simulink model "lab02_Digital_Inputs_and_Outputs"  (R2022b)
settings: Solver=FixedStepAuto  StartTime=0.0  StopTime=inf  RelTol=1e-3
libraries: arduinolib x10, simulink x6
settings Model: ExtModeTrigDuration=2  Creator=MAAM  LastModifiedBy=MAAM
settings OptimizationCC: EnhancedBackFolding=on  PassReuseOutputArgsAs=Individual arguments  ZeroExternalMemoryAtStartup=off  ZeroInternalMemoryAtStartup=off  MaxStackSize=64  OptimizeBlockOrder=speed  DifferentSizesBufferReuse=on  OptimizationCustomize=off  EfficientTunableParamExpr=on
settings DebuggingCC: ParameterTunabilityLossMsg=error
settings HardwareCC: ProdBitPerInt=16  ProdBitPerPointer=16  ProdBitPerSizeT=16  ProdBitPerPtrDiffT=16  ProdLargestAtomicFloat=None  ProdWordSize=8  ProdHWDeviceType=Atmel->AVR
settings SFSimCC: MATLABDynamicMemAlloc=off
settings RTWCC: Description=Embedded Coder  SystemTargetFile=ert.tlc  HardwareBoard=Arduino Mega 2560  TemplateMakefile=ert_default_tmf  Toolchain=Arduino AVR  BuildConfiguration=Faster Runs
settings CodeAppCC: ForceParamTrailComments=on  IgnoreCustomStorageClasses=off  OperatorAnnotations=on  SimulinkDataObjDesc=on  SFDataObjDesc=on  InsertBlockDesc=on
settings ERTTargetCC: SupportContinuousTime=on  SupportVariableSizeSignals=on  ExtMode=on  ExtModeTransport=3  ExtModeStaticAlloc=on  ExtModeAutomaticAllocSize=off  ExtModeStaticAllocSize=2048  ExtModeMexFile=ext_xcp  ExtModeMexArgs=0 5 921600  ExtModeIntrfLevel=Level2 - Open

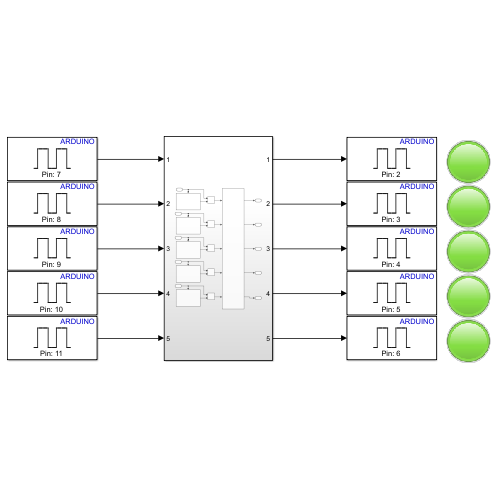
[thumbnail: Simulink's stored preview of the top-level diagram]
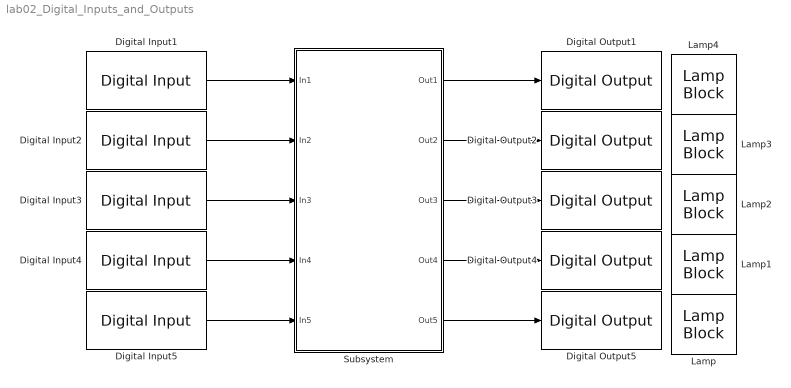
== system lab02_Digital_Inputs_and_Outputs ==
  Digital Input1 : arduinolib/Digital Input  pinNumber=7  mode=Default  Direction=input  SampleTime=-1  blockPlatform=arduino
  Digital Input2 : arduinolib/Digital Input  pinNumber=8  mode=Default  Direction=input  SampleTime=-1  blockPlatform=arduino
  Digital Input3 : arduinolib/Digital Input  pinNumber=9  mode=Default  Direction=input  SampleTime=-1  blockPlatform=arduino
  Digital Input4 : arduinolib/Digital Input  pinNumber=10  mode=Default  Direction=input  SampleTime=-1  blockPlatform=arduino
  Digital Input5 : arduinolib/Digital Input  pinNumber=11  mode=Default  Direction=input  SampleTime=-1  blockPlatform=arduino
  Digital Output1 : arduinolib/Digital Output  pinNumber=2  Direction=output  blockPlatform=arduino
  Digital Output2 : arduinolib/Digital Output  pinNumber=3  Direction=output  blockPlatform=arduino
  Digital Output3 : arduinolib/Digital Output  pinNumber=4  Direction=output  blockPlatform=arduino
  Digital Output4 : arduinolib/Digital Output  pinNumber=5  Direction=output  blockPlatform=arduino
  Digital Output5 : arduinolib/Digital Output  pinNumber=6  Direction=output  blockPlatform=arduino
  Lamp{,1..4} (5 alike) : LampBlock  LabelPosition=Hide
  Subsystem : Subsystem
  wires:
  Subsystem/4(Out4) -> Digital Output4/1
  Subsystem/3(Out3) -> Digital Output3/1
  Subsystem/2(Out2) -> Digital Output2/1
  Subsystem/1(Out1) -> Digital Output1/1
  Digital Input1/1 -> Subsystem/1(In1)
  Digital Input2/1 -> Subsystem/2(In2)
  Digital Input3/1 -> Subsystem/3(In3)
  Digital Input4/1 -> Subsystem/4(In4)
  Digital Input5/1 -> Subsystem/5(In5)
  Subsystem/5(Out5) -> Digital Output5/1

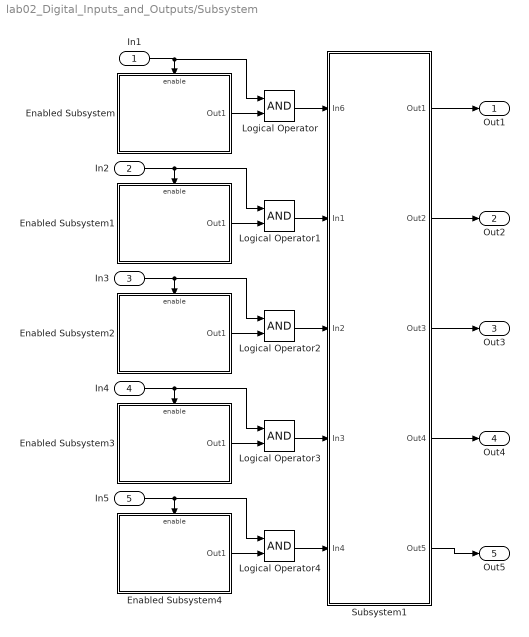
== system lab02_Digital_Inputs_and_Outputs/Subsystem ==
  In1 : Inport
  In2 : Inport  Port=2
  In3 : Inport  Port=3
  In4 : Inport  Port=4
  In5 : Inport  Port=5
  Enabled Subsystem : Subsystem  TreatAsAtomicUnit=on
  Enabled Subsystem1 : Subsystem  TreatAsAtomicUnit=on
  Enabled Subsystem2 : Subsystem  TreatAsAtomicUnit=on
  Enabled Subsystem3 : Subsystem  TreatAsAtomicUnit=on
  Enabled Subsystem4 : Subsystem  TreatAsAtomicUnit=on
  Logical Operator{,1..4} (5 alike) : Logic  AllPortsSameDT=off  OutDataTypeStr=boolean
  Subsystem1 : Subsystem
  Out1 : Outport
  Out2 : Outport  Port=2
  Out3 : Outport  Port=3
  Out4 : Outport  Port=4
  Out5 : Outport  Port=5
  wires:
  In1/1 -> Logical Operator/1, Enabled Subsystem/Enable
  In2/1 -> Logical Operator1/1, Enabled Subsystem1/Enable
  In3/1 -> Enabled Subsystem2/Enable, Logical Operator2/1
  In4/1 -> Logical Operator3/1, Enabled Subsystem3/Enable
  In5/1 -> Logical Operator4/1, Enabled Subsystem4/Enable
  Enabled Subsystem/1(Out1) -> Logical Operator/2
  Enabled Subsystem1/1(Out1) -> Logical Operator1/2
  Enabled Subsystem2/1(Out1) -> Logical Operator2/2
  Enabled Subsystem3/1(Out1) -> Logical Operator3/2
  Enabled Subsystem4/1(Out1) -> Logical Operator4/2
  Subsystem1/5(Out5) -> Out5/1
  Subsystem1/4(Out4) -> Out4/1
  Subsystem1/3(Out3) -> Out3/1
  Subsystem1/2(Out2) -> Out2/1
  Subsystem1/1(Out1) -> Out1/1
  Logical Operator4/1 -> Subsystem1/5(In4)
  Logical Operator3/1 -> Subsystem1/4(In3)
  Logical Operator2/1 -> Subsystem1/3(In2)
  Logical Operator1/1 -> Subsystem1/2(In1)
  Logical Operator/1 -> Subsystem1/1(In6)

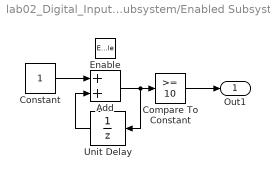
== system lab02_Digital_Inputs_and_Outputs/Subsystem/Enabled Subsystem ==
  Enable : EnablePort  StatesWhenEnabling=reset
  Add : Sum
  Compare To Constant : simulink/Logic and Bit Operations/Compare To Constant  relop=>=  const=10  OutDataTypeStr=boolean
  Constant : Constant
  Unit Delay : UnitDelay  SampleTime=0.1  HasFrameUpgradeWarning=on
  Out1 : Outport
  wires:
  Add/1 -> Compare To Constant/1, Unit Delay/1
  Unit Delay/1 -> Add/2
  Constant/1 -> Add/1
  Compare To Constant/1 -> Out1/1

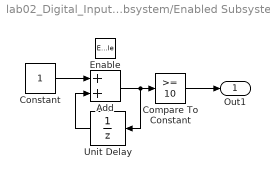
== system lab02_Digital_Inputs_and_Outputs/Subsystem/Enabled Subsystem1 ==
  Enable : EnablePort  StatesWhenEnabling=reset
  Add : Sum
  Compare To Constant : simulink/Logic and Bit Operations/Compare To Constant  relop=>=  const=10  OutDataTypeStr=boolean
  Constant : Constant
  Unit Delay : UnitDelay  SampleTime=0.1  HasFrameUpgradeWarning=on
  Out1 : Outport
  wires:
  Compare To Constant/1 -> Out1/1
  Constant/1 -> Add/1
  Unit Delay/1 -> Add/2
  Add/1 -> Unit Delay/1, Compare To Constant/1

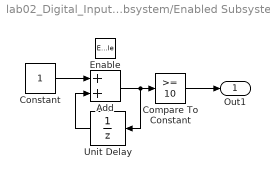
== system lab02_Digital_Inputs_and_Outputs/Subsystem/Enabled Subsystem2 ==
  Enable : EnablePort  StatesWhenEnabling=reset
  Add : Sum
  Compare To Constant : simulink/Logic and Bit Operations/Compare To Constant  relop=>=  const=10  OutDataTypeStr=boolean
  Constant : Constant
  Unit Delay : UnitDelay  SampleTime=0.1  HasFrameUpgradeWarning=on
  Out1 : Outport
  wires:
  Add/1 -> Compare To Constant/1, Unit Delay/1
  Unit Delay/1 -> Add/2
  Constant/1 -> Add/1
  Compare To Constant/1 -> Out1/1

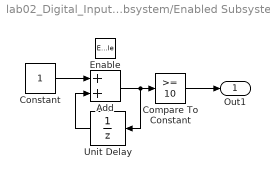
== system lab02_Digital_Inputs_and_Outputs/Subsystem/Enabled Subsystem3 ==
  Enable : EnablePort  StatesWhenEnabling=reset
  Add : Sum
  Compare To Constant : simulink/Logic and Bit Operations/Compare To Constant  relop=>=  const=10  OutDataTypeStr=boolean
  Constant : Constant
  Unit Delay : UnitDelay  SampleTime=0.1  HasFrameUpgradeWarning=on
  Out1 : Outport
  wires:
  Compare To Constant/1 -> Out1/1
  Constant/1 -> Add/1
  Unit Delay/1 -> Add/2
  Add/1 -> Unit Delay/1, Compare To Constant/1

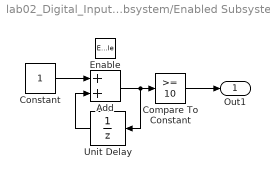
== system lab02_Digital_Inputs_and_Outputs/Subsystem/Enabled Subsystem4 ==
  Enable : EnablePort  StatesWhenEnabling=reset
  Add : Sum
  Compare To Constant : simulink/Logic and Bit Operations/Compare To Constant  relop=>=  const=10  OutDataTypeStr=boolean
  Constant : Constant
  Unit Delay : UnitDelay  SampleTime=0.1  HasFrameUpgradeWarning=on
  Out1 : Outport
  wires:
  Add/1 -> Compare To Constant/1, Unit Delay/1
  Unit Delay/1 -> Add/2
  Constant/1 -> Add/1
  Compare To Constant/1 -> Out1/1

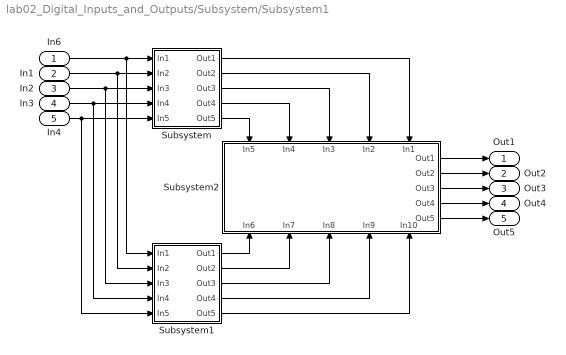
== system lab02_Digital_Inputs_and_Outputs/Subsystem/Subsystem1 ==
  In6 : Inport
  In1 : Inport  Port=2
  In2 : Inport  Port=3
  In3 : Inport  Port=4
  In4 : Inport  Port=5
  Subsystem : Subsystem
  Subsystem1 : Subsystem
  Subsystem2 : Subsystem
      settings: PortSchema="{\"entries\":[{\"content\":{\"sides\":[{\"content\":{\"connectorIds\":[]},\"type\":\"ConnectorPlacement.EquallySpacedRectSide\",\"uuid\":\"3d5a28fc-197f-44ec-9451-d26fad6cf1b4\"},{\"content\":{\"connectorIds\":[\"Out1\",\"Out2\",\"Out3\",\"Out4\",\"Out5\"],\"side\":\"RIGHT\"},\"type\":\"ConnectorPlacement.EquallySpacedRectSide\",\"uuid\":\"92fd3327-f770-4999-b898-3eaeca0147e0\"},{\"content\":{\"connectorIds\":[\"In1\",\"In2\",\"In3\",\"In4\",\"In5\"],\"side\":\"TOP\"},\"type\":\"ConnectorPlacement.EquallySpacedRectSide\",\"uuid\":\"be5c574c-d851-45a7-98e5-1ded246edbd4\"},{\"content\":{\"connectorIds\":[\"In6\",\"In7\",\"In8\",\"In9\",\"In10\"],\"side\":\"BOTTOM\"},\"type\":\"ConnectorPlacement.EquallySpacedRectSide\",\"uuid\":\"0069f3dc-259c-45b3-8447-ee377a9961bb\"}]},\"type\":\"ConnectorPlacement.EquallySpacedConnector\",\"uuid\":\"4cce2df6-098f-4a42-be6d-81f6fd067375\"}],\"packageUris\":[\"http://schema.mathworks.com/mf0/Connector/R2020b\"],\"version\":\"1.0\"}"
  Out1 : Outport
  Out2 : Outport  Port=2
  Out3 : Outport  Port=3
  Out4 : Outport  Port=4
  Out5 : Outport  Port=5
  wires:
  In6/1 -> Subsystem1/1(In1), Subsystem/1(In1)
  In1/1 -> Subsystem1/2(In2), Subsystem/2(In2)
  In2/1 -> Subsystem1/3(In3), Subsystem/3(In3)
  In3/1 -> Subsystem/4(In4), Subsystem1/4(In4)
  In4/1 -> Subsystem1/5(In5), Subsystem/5(In5)
  Subsystem/1(Out1) -> Subsystem2/5(In1)
  Subsystem/2(Out2) -> Subsystem2/4(In2)
  Subsystem/3(Out3) -> Subsystem2/3(In3)
  Subsystem/4(Out4) -> Subsystem2/2(In4)
  Subsystem/5(Out5) -> Subsystem2/1(In5)
  Subsystem1/1(Out1) -> Subsystem2/6(In6)
  Subsystem1/2(Out2) -> Subsystem2/7(In7)
  Subsystem1/3(Out3) -> Subsystem2/8(In8)
  Subsystem1/4(Out4) -> Subsystem2/9(In9)
  Subsystem1/5(Out5) -> Subsystem2/10(In10)
  Subsystem2/1(Out1) -> Out1/1
  Subsystem2/2(Out2) -> Out2/1
  Subsystem2/3(Out3) -> Out3/1
  Subsystem2/4(Out4) -> Out4/1
  Subsystem2/5(Out5) -> Out5/1

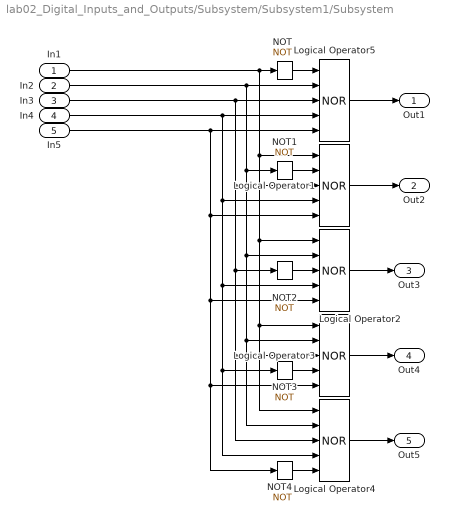
== system lab02_Digital_Inputs_and_Outputs/Subsystem/Subsystem1/Subsystem ==
  In1 : Inport
  In2 : Inport  Port=2
  In3 : Inport  Port=3
  In4 : Inport  Port=4
  In5 : Inport  Port=5
  Logical Operator{1..5} (5 alike) : Logic  Operator=NOR  Inputs=5  AllPortsSameDT=off  OutDataTypeStr=boolean
  NOT{,1..4} (5 alike) : Logic  Operator=NOT  IconShape=distinctive  AllPortsSameDT=off  OutDataTypeStr=boolean
  Out1 : Outport
  Out2 : Outport  Port=2
  Out3 : Outport  Port=3
  Out4 : Outport  Port=4
  Out5 : Outport  Port=5
  wires:
  In3/1 -> Logical Operator1/3, NOT2/1, Logical Operator4/3, Logical Operator3/3, Logical Operator5/3
  NOT3/1 -> Logical Operator3/4
  In1/1 -> Logical Operator4/1, Logical Operator3/1, Logical Operator2/1, Logical Operator1/1, NOT/1
  NOT1/1 -> Logical Operator1/2
  In5/1 -> Logical Operator1/5, Logical Operator2/5, Logical Operator3/5, NOT4/1, Logical Operator5/5
  In2/1 -> Logical Operator5/2, NOT1/1, Logical Operator2/2, Logical Operator3/2, Logical Operator4/2
  In4/1 -> Logical Operator1/4, Logical Operator2/4, NOT3/1, Logical Operator4/4, Logical Operator5/4
  Logical Operator4/1 -> Out5/1
  NOT/1 -> Logical Operator5/1
  Logical Operator3/1 -> Out4/1
  NOT4/1 -> Logical Operator4/5
  Logical Operator2/1 -> Out3/1
  NOT2/1 -> Logical Operator2/3
  Logical Operator1/1 -> Out2/1
  Logical Operator5/1 -> Out1/1

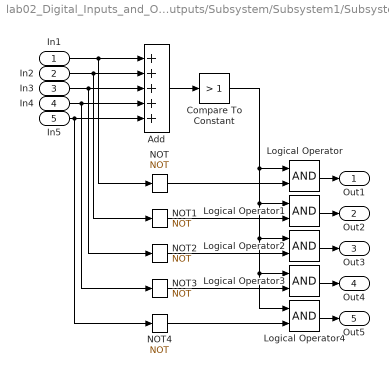
== system lab02_Digital_Inputs_and_Outputs/Subsystem/Subsystem1/Subsystem1 ==
  In1 : Inport
  In2 : Inport  Port=2
  In3 : Inport  Port=3
  In4 : Inport  Port=4
  In5 : Inport  Port=5
  Add : Sum  Inputs=+++++
  Compare To Constant : simulink/Logic and Bit Operations/Compare To Constant  relop=>  const=1  OutDataTypeStr=boolean
  Logical Operator{,1..4} (5 alike) : Logic  AllPortsSameDT=off  OutDataTypeStr=boolean
  NOT{,1..4} (5 alike) : Logic  Operator=NOT  IconShape=distinctive  AllPortsSameDT=off  OutDataTypeStr=boolean
  Out1 : Outport
  Out2 : Outport  Port=2
  Out3 : Outport  Port=3
  Out4 : Outport  Port=4
  Out5 : Outport  Port=5
  wires:
  In1/1 -> NOT/1, Add/1
  In2/1 -> NOT1/1, Add/2
  In3/1 -> NOT2/1, Add/3
  In4/1 -> NOT3/1, Add/4
  In5/1 -> NOT4/1, Add/5
  Add/1 -> Compare To Constant/1
  Logical Operator/1 -> Out1/1
  Compare To Constant/1 -> Logical Operator2/1, Logical Operator3/1, Logical Operator4/1, Logical Operator1/1, Logical Operator/1
  Logical Operator1/1 -> Out2/1
  Logical Operator2/1 -> Out3/1
  Logical Operator4/1 -> Out5/1
  Logical Operator3/1 -> Out4/1
  NOT/1 -> Logical Operator/2
  NOT1/1 -> Logical Operator1/2
  NOT2/1 -> Logical Operator2/2
  NOT3/1 -> Logical Operator3/2
  NOT4/1 -> Logical Operator4/2

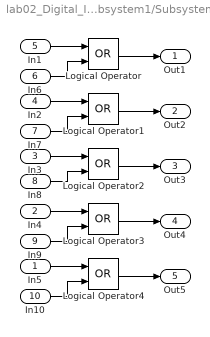
== system lab02_Digital_Inputs_and_Outputs/Subsystem/Subsystem1/Subsystem2 ==
  In5 : Inport
  In4 : Inport  Port=2
  In3 : Inport  Port=3
  In2 : Inport  Port=4
  In1 : Inport  Port=5
  In6 : Inport  Port=6
  In7 : Inport  Port=7
  In8 : Inport  Port=8
  In9 : Inport  Port=9
  In10 : Inport  Port=10
  Logical Operator{,1..4} (5 alike) : Logic  Operator=OR  AllPortsSameDT=off  OutDataTypeStr=boolean
  Out1 : Outport
  Out2 : Outport  Port=2
  Out3 : Outport  Port=3
  Out4 : Outport  Port=4
  Out5 : Outport  Port=5
  wires:
  In5/1 -> Logical Operator4/1
  In6/1 -> Logical Operator/2
  In10/1 -> Logical Operator4/2
  In9/1 -> Logical Operator3/2
  In2/1 -> Logical Operator1/1
  In1/1 -> Logical Operator/1
  In3/1 -> Logical Operator2/1
  In8/1 -> Logical Operator2/2
  In4/1 -> Logical Operator3/1
  In7/1 -> Logical Operator1/2
  Logical Operator4/1 -> Out5/1
  Logical Operator/1 -> Out1/1
  Logical Operator2/1 -> Out3/1
  Logical Operator3/1 -> Out4/1
  Logical Operator1/1 -> Out2/1
